simulink model "linearise_model2"  (R2021b)
settings: Solver=VariableStepAuto  StartTime=0.0  StopTime=100  RelTol=1e-3
values from neighbouring files (symbols this model uses):
  alpha = 3.7541    [Parameters.m]
  beta = beta/(24*60*60)    (= 1.57476851852e-05)    [Parameters.m]
  dI = dI/(24*60*60)    (= 1.15740740741e-06)    [Parameters.m]
  dV = dV/(24*60*60)    (= 2.13148148148e-05)    [Parameters.m]
  I0 = 0    [Parameters.m]
  L = 936.4293    [Parameters.m]
  r = r/(24*60*60)    (= 6.97916666667e-07)    [Parameters.m]
  S0 = 128.1481    [Parameters.m]
  V0 = 0    [Parameters.m]
settings Model: Creator=zceexc1  LastModifiedBy=chenx
settings DebuggingCC: UnconnectedInputMsg=none  UnconnectedOutputMsg=none  UnconnectedLineMsg=none
settings RTWCC: DLArmComputeVersion=20.02.1

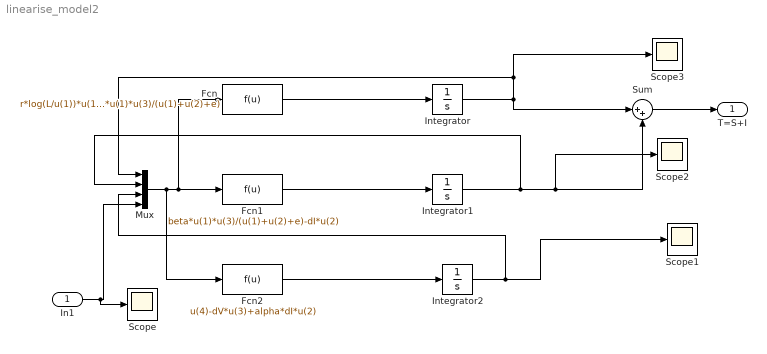
== system linearise_model2 ==
  In1 : Inport
  Fcn : Fcn  Expr=r*log(L/u(1))*u(1)-beta*u(1)*u(3)/(u(1)+u(2)+e)
  Fcn1 : Fcn  Expr=beta*u(1)*u(3)/(u(1)+u(2)+e)-dI*u(2)
  Fcn2 : Fcn  Expr=u(4)-dV*u(3)+alpha*dI*u(2)
  Integrator : Integrator  InitialCondition=S0
  Integrator1 : Integrator  InitialCondition=I0
  Integrator2 : Integrator  InitialCondition=V0
  Mux : Mux
  Scope{,1..3} (4 alike) : Scope
  Sum : Sum  Inputs=|++
  T=S+I : Outport
  wires:
  Fcn/1 -> Integrator/1
  Fcn1/1 -> Integrator1/1
  Fcn2/1 -> Integrator2/1
  Integrator2/1 -> Mux/3, Scope1/1
  Integrator/1 -> Sum/1, Scope3/1, Mux/1
  Integrator1/1 -> Sum/2, Scope2/1, Mux/2
  Mux/1 -> Fcn2/1, Fcn1/1, Fcn/1
  In1/1 -> Mux/4, Scope/1
  Sum/1 -> T=S+I/1
